simulink model "Copy_of_kalman_estimate"  (R2018b)
settings: Solver=FixedStepAuto  StartTime=0.0  StopTime=2000  FixedStep=0.02  RelTol=1e-3
undefined symbols (not defined in the file or in its folder): Discrete, piece, Time
libraries: sharedschedule x15, commchan3 x1, ctrlSharedLib x1, simulink x1
settings Model: Creator=mmm  LastModifiedBy=mmm

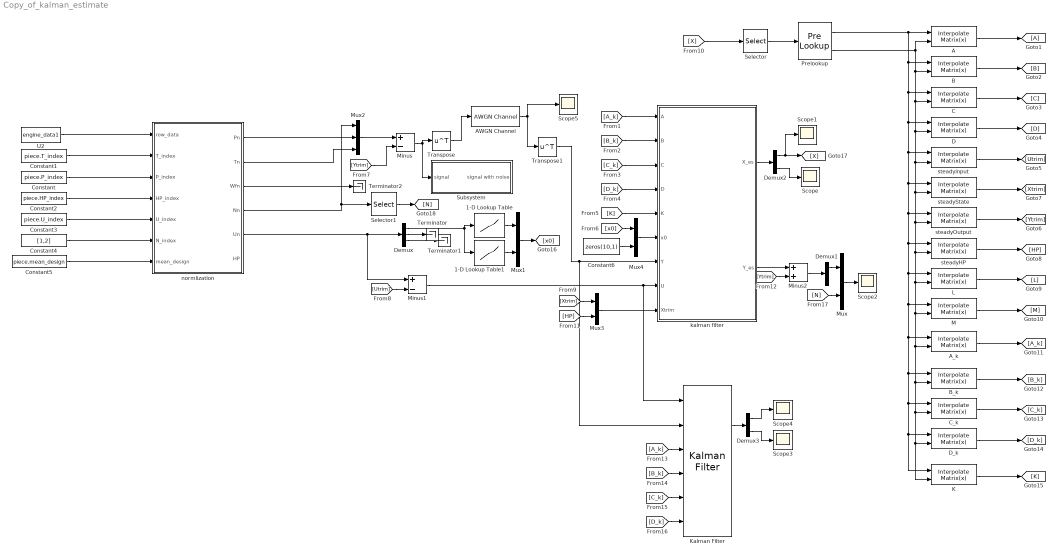
== system Copy_of_kalman_estimate ==
  1-D Lookup Table : Lookup_n-D  NumberOfTableDimensions=1  BreakpointsForDimension1=piece.Wf_stable_(:,1)  Table=piece.Nl  InterpMethod=Cubic spline  ExtrapMethod=Cubic spline  InternalRulePriority=Speed  RndMeth=Simplest  InputSameDT=on
  1-D Lookup Table1 : Lookup_n-D  NumberOfTableDimensions=1  BreakpointsForDimension1=piece.Wf_stable_(:,1)  Table=piece.N_stable_(:,2)  InterpMethod=Cubic spline  ExtrapMethod=Cubic spline  InternalRulePriority=Speed  RndMeth=Simplest  InputSameDT=on
  A : sharedschedule/Interpolate Matrix(x)   matrix=piece.A  aMode=aMode
      settings: SourceProductName=Aerospace Blockset  SourceProductBaseCode=AE
  AWGN Channel : commchan3/AWGN Channel  InputProcessing=Columns as channels (frame based)  seed=11:20  noiseMode=Variance from mask  EbNodB=10  EsNodB=10  SNRdB=10  bitsPerSym=1  Ps=1  Tsym=1  variance=[0.0025,0.0025,0.005,0.005,0.005,0.005,0.0075,0.0075,0.0075,0.0075].^2
  A_k : sharedschedule/Interpolate Matrix(x)   matrix=piece.A_k  aMode=aMode
      settings: SourceProductName=Aerospace Blockset  SourceProductBaseCode=AE
  B : sharedschedule/Interpolate Matrix(x)   matrix=piece.B  aMode=aMode
      settings: SourceProductName=Aerospace Blockset  SourceProductBaseCode=AE
  B_k : sharedschedule/Interpolate Matrix(x)   matrix=piece.B_k  aMode=aMode
      settings: SourceProductName=Aerospace Blockset  SourceProductBaseCode=AE
  C : sharedschedule/Interpolate Matrix(x)   matrix=piece.C  aMode=aMode
      settings: SourceProductName=Aerospace Blockset  SourceProductBaseCode=AE
  C_k : sharedschedule/Interpolate Matrix(x)   matrix=piece.C_k  aMode=aMode
      settings: SourceProductName=Aerospace Blockset  SourceProductBaseCode=AE
  Constant : Constant  Value=piece.P_index  VectorParams1D=off
  Constant1 : Constant  Value=piece.T_index  VectorParams1D=off
  Constant2 : Constant  Value=piece.HP_index  VectorParams1D=off
  Constant3 : Constant  Value=piece.U_index  VectorParams1D=off
  Constant4 : Constant  Value=[1,2]  VectorParams1D=off
  Constant5 : Constant  Value=piece.mean_design  VectorParams1D=off
  Constant6 : Constant  Value=zeros(10,1)  VectorParams1D=off
  D : sharedschedule/Interpolate Matrix(x)   matrix=piece.D  aMode=aMode
      settings: SourceProductName=Aerospace Blockset  SourceProductBaseCode=AE
  D_k : sharedschedule/Interpolate Matrix(x)   matrix=piece.D_k  aMode=aMode
      settings: SourceProductName=Aerospace Blockset  SourceProductBaseCode=AE
  Demux : Demux  Outputs=3
  Demux1 : Demux  Outputs=[1,1,8]
  Demux2 : Demux  Outputs=[2,10]
  Demux3 : Demux  Outputs=[2,10]
  K : sharedschedule/Interpolate Matrix(x)   matrix=piece.K  aMode=aMode
      settings: SourceProductName=Aerospace Blockset  SourceProductBaseCode=AE
  Kalman Filter : ctrlSharedLib/Kalman Filter  TimeDomain=Discrete-Time  UseCurrentEstimator=on  ModelSource=Input port  ModelSourceVariable=ss(0.95,1,1,0,1)  A=0.95  B=1  C=1  D=0  NumberOfStates=12  NumberOfInputs=3  NumberOfOutputs=10  InitialEstimateSource=Dialog  X0=0  P0=0.1  UseK=off  UseGH=off  NumberOfProcessNoiseInputs=1  G=1  TimeInvariantG=on  H=0  TimeInvariantH=on  Q=0.0002^2  TimeInvariantQ=on  R=[0.0025,0.0025,0.005,0.005,0.005,0.005,0.0075,0.0075,0.0075,0.0075].^2  TimeInvariantR=on  N=0  TimeInvariantN=on  AddInputPort=on  AddEnablePort=off  OutputEstimatedY=on  OutputP=off  Ts=-1
      settings: SourceProductBaseCode=CT
  L : sharedschedule/Interpolate Matrix(x)   matrix=piece.L  aMode=aMode
      settings: SourceProductName=Aerospace Blockset  SourceProductBaseCode=AE
  M : sharedschedule/Interpolate Matrix(x)   matrix=piece.M  aMode=aMode
      settings: SourceProductName=Aerospace Blockset  SourceProductBaseCode=AE
  Minus : Sum  Inputs=+-
  Minus1 : Sum  Inputs=+-
  Minus2 : Sum
  Mux{,1,3..4} (4 alike) : Mux  Inputs=2
  Mux2 : Mux  Inputs=3
  Prelookup : PreLookup  BreakpointsData=piece.Nl  BreakpointObject=Nl  ExtrapMethod=Linear  UseLastBreakpoint=on  DiagnosticForOutOfRangeInput=Warning
  Scope{,1..5} (6 alike) : Scope
  Selector : Selector  InputPortWidth=2  IndexOptions=Index vector (dialog)  Indices=[1]  OutputSizes=1
  Selector1 : Selector  InputPortWidth=2  IndexOptions=Index vector (dialog)  Indices=[1]  OutputSizes=1
  Subsystem : Subsystem
  Terminator : Terminator
  Terminator1 : Terminator
  Terminator2 : Terminator
  Transpose : Math  Operator=transpose  SaturateOnIntegerOverflow=on
  Transpose1 : Math  Operator=transpose  SaturateOnIntegerOverflow=on
  U2 : FromWorkspace  VariableName=engine_data1  SampleTime=0.02  Interpolate=off  OutputAfterFinalValue=Holding final value
  kalman filter : Subsystem
  normlization : MATLAB Function  TreatAsAtomicUnit=on
  steadyHP : sharedschedule/Interpolate Matrix(x)   matrix=piece.steadyHP  aMode=aMode
      settings: SourceProductName=Aerospace Blockset  SourceProductBaseCode=AE
  steadyOutput : sharedschedule/Interpolate Matrix(x)   matrix=piece.steadyOutput  aMode=aMode
      settings: SourceProductName=Aerospace Blockset  SourceProductBaseCode=AE
  steadyState : sharedschedule/Interpolate Matrix(x)   matrix=piece.steadyState  aMode=aMode
      settings: SourceProductName=Aerospace Blockset  SourceProductBaseCode=AE
  steadyinput : sharedschedule/Interpolate Matrix(x)   matrix=piece.steadyInput  aMode=aMode
      settings: SourceProductName=Aerospace Blockset  SourceProductBaseCode=AE
  wires:
  Constant4/1 -> normlization/6(N_index)
  Constant2/1 -> normlization/4(HP_index)
  Constant3/1 -> normlization/5(U_index)
  Constant1/1 -> normlization/2(T_index)
  Constant5/1 -> normlization/7(mean_design)
  normlization/3(Wfn) -> Terminator2/1
  U2/1 -> normlization/1(row_data)
  Constant/1 -> normlization/3(P_index)
  K/1 -> [K]
  B_k/1 -> [B_k]
  C_k/1 -> [C_k]
  D_k/1 -> [D_k]
  A_k/1 -> [A_k]
  steadyinput/1 -> [Utrim]
  [X] -> Selector/1
  Prelookup/2 -> A/2, steadyState/2, steadyOutput/2, steadyHP/2, L/2, B_k/2, C_k/2, K/2, D_k/2, A_k/2, M/2, steadyinput/2, D/2, C/2, B/2
  steadyState/1 -> [Xtrim]
  B/1 -> [B]
  steadyHP/1 -> [HP]
  steadyOutput/1 -> [Ytrim]
  D/1 -> [D]
  A/1 -> [A]
  C/1 -> [C]
  L/1 -> [L]
  M/1 -> [M]
  Prelookup/1 -> steadyState/1, steadyOutput/1, steadyHP/1, L/1, B_k/1, C_k/1, K/1, D_k/1, A_k/1, M/1, steadyinput/1, D/1, C/1, B/1, A/1
  Selector/1 -> Prelookup/1
  [A_k] -> kalman filter/1(A)
  [B_k] -> kalman filter/2(B)
  [C_k] -> kalman filter/3(C)
  [D_k] -> kalman filter/4(D)
  [K] -> kalman filter/5(K)
  normlization/5(Un) -> Minus1/1, Demux/1
  Demux/1 -> 1-D Lookup Table1/1, 1-D Lookup Table/1
  Demux/2 -> Terminator/1
  Demux/3 -> Terminator1/1
  1-D Lookup Table/1 -> Mux1/1
  1-D Lookup Table1/1 -> Mux1/2
  Mux1/1 -> [x0]
  Mux2/1 -> Minus/1
  [Ytrim] -> Minus/2
  [Utrim] -> Minus1/2
  Minus1/1 -> Kalman Filter/1, kalman filter/8(U)
  Minus/1 -> Subsystem/1(signal), Transpose/1
  [Xtrim] -> Mux3/1
  [HP] -> Mux3/2
  Mux3/1 -> kalman filter/9(Xtrim)
  kalman filter/1(X_es) -> Demux2/1
  Demux2/1 -> Scope1/1, [X]
  [x0] -> Mux4/1
  Constant6/1 -> Mux4/2
  Mux4/1 -> kalman filter/6(x0)
  normlization/1(Pn) -> Mux2/2
  normlization/2(Tn) -> Mux2/3
  normlization/4(Nn) -> Mux2/1, Selector1/1
  kalman filter/2(Y_es) -> Minus2/1
  [Ytrim] -> Minus2/2
  Minus2/1 -> Demux1/1
  [A_k] -> Kalman Filter/3
  [B_k] -> Kalman Filter/4
  [C_k] -> Kalman Filter/5
  [D_k] -> Kalman Filter/6
  Demux3/2 -> Scope3/1
  Demux3/1 -> Scope4/1
  Kalman Filter/1 -> Demux3/1
  Demux1/1 -> Mux/1
  Selector1/1 -> [N]
  [N] -> Mux/2
  Mux/1 -> Scope2/1
  AWGN Channel/1 -> Transpose1/1, Scope5/1
  Transpose/1 -> AWGN Channel/1
  Transpose1/1 -> kalman filter/7(Y), Kalman Filter/2
  Demux2/2 -> Scope/1

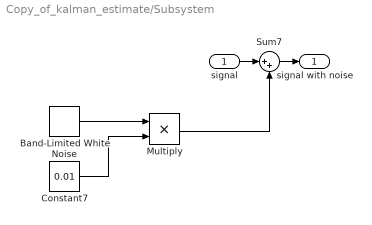
== system Copy_of_kalman_estimate/Subsystem ==
  signal : Inport
  Band-Limited White Noise : simulink/Sources/Band-Limited White Noise  Cov=ones(10,1)*0.0025^2*0.02  Ts=0.02  seed=[1000:500:5500]
  Constant7 : Constant  Value=0.01
  Multiply : Product
  Sum7 : Sum  Inputs=|++
  signal with noise : Outport
  wires:
  Constant7/1 -> Multiply/2
  Multiply/1 -> Sum7/2
  signal/1 -> Sum7/1
  Sum7/1 -> signal with noise/1
  Band-Limited White Noise/1 -> Multiply/1

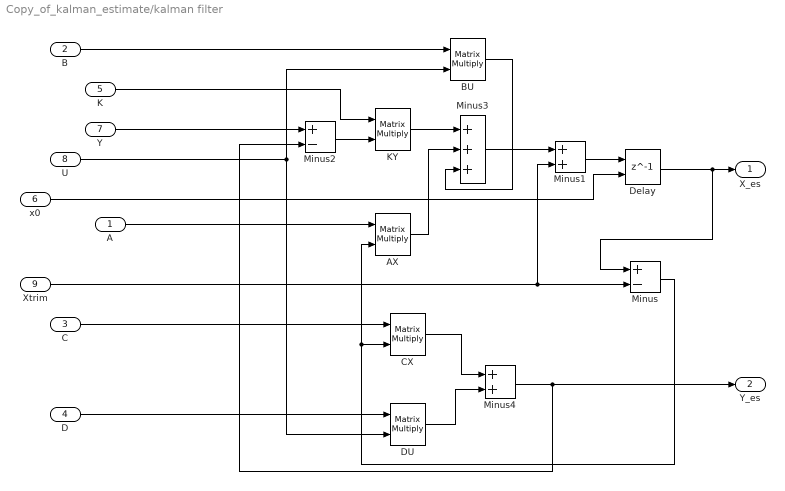
== system Copy_of_kalman_estimate/kalman filter ==
  A : Inport
  B : Inport  Port=2
  C : Inport  Port=3
  D : Inport  Port=4
  K : Inport  Port=5
  x0 : Inport  Port=6
  Y : Inport  Port=7
  U : Inport  Port=8
  Xtrim : Inport  Port=9
  "\tCX" : Product  Multiplication=Matrix(*)
  AX : Product  Multiplication=Matrix(*)
  BU : Product  Multiplication=Matrix(*)
  DU : Product  Multiplication=Matrix(*)
  Delay : Delay  DelayLength=1  InitialConditionSource=Input port
      settings: InputPortMap=u0,p4
  KY : Product  Multiplication=Matrix(*)
  Minus : Sum  Inputs=+-
  Minus1 : Sum
  Minus2 : Sum  Inputs=+-
  Minus3 : Sum  Inputs=+++
  Minus4 : Sum
  X_es : Outport
  Y_es : Outport  Port=2
  wires:
  Minus4/1 -> Minus2/2, Y_es/1
  KY/1 -> Minus3/1
  U/1 -> BU/2, DU/2
  Y/1 -> Minus2/1
  DU/1 -> Minus4/2
  "\tCX"/1 -> Minus4/1
  x0/1 -> Delay/2
  Minus2/1 -> KY/2
  BU/1 -> Minus3/3
  A/1 -> AX/1
  B/1 -> BU/1
  C/1 -> "\tCX"/1
  D/1 -> DU/1
  K/1 -> KY/1
  Xtrim/1 -> Minus1/2, Minus/2
  Delay/1 -> Minus/1, X_es/1
  Minus/1 -> AX/2, "\tCX"/2
  AX/1 -> Minus3/2
  Minus3/1 -> Minus1/1
  Minus1/1 -> Delay/1

== matlab function Copy_of_kalman_estimate/normlization ==
  data: Pn output; row_data input; Tn output; T_index input; P_index input; HP_index input; U_index input; N_index input; mean_design input; Wfn output; Nn output; Un output; HP output
function [Pn,Tn,Wfn,Nn,Un,HP] = fcn(row_data,T_index,P_index,HP_index,U_index,N_index,mean_design)
%%% 数据相似归一化
if size(mean_design,1) > size(mean_design,2)
    mean_ = mean_design';
else
    mean_ = mean_design;
end
if size(T_index,1) > size(T_index,2)
    T_index_ = T_index';
else
    T_index_ = T_index;
end
if size(P_index,1) > size(P_index,2)
    P_index_ = P_index';
else
    P_index_ = P_index;
end
if size(HP_index,1) > size(HP_index,2)
    HP_index_ = HP_index';
else
    HP_index_ = HP_index;
end
if size(U_index,1) > size(U_index,2)
    U_index_ = U_index';
else
    U_index_ = U_index;
end
if size(N_index,1) > size(N_index,2)
    N_index_ = N_index';
else
    N_index_ = N_index;
end
if size(row_data,1)>size(row_data,2)
    row = row_data';
else
    row = row_data;
end
T2_index = 12;
P2_index = 13;
T = row(:,T_index_);
P = row(:,P_index_);
HP = row(:,HP_index_)'-1;
U = row(:,U_index_);
N = row(:,N_index_);
sigma_P = mean_(P_index_)./mean_(P2_index);
sigma_T = mean_(T_index_)./mean_(T2_index);
sigma_Wf = mean_(U_index_(:,1)).*sqrt(mean_(T2_index))./mean_(P2_index);
sigma_N = mean_(N_index_)./mean_(T2_index);
Tn = [(T./row(:,T2_index))./sigma_T]';
Pn = [(P./row(:,P2_index))./sigma_P]';
Wfn = (U(:,1).*sqrt(row(:,T2_index))./row(:,P2_index))./sigma_Wf;
Nn = [N./row(:,T2_index)./sigma_N]';
Un = [Wfn,U(:,2:end)]';
